simulink model "p1"  (R2014a)
settings: Solver=ode1  SolverMode=SingleTasking  StartTime=0  StopTime=36000  FixedStep=Ts  RelTol=1e-3
PreLoadFcn:
  | InitModel
  | make
InitFcn:
  | InitModel
  | make
values from neighbouring files (symbols this model uses):
  num = num+MTnum(m)    [Build_MtMuMy.m]
  Ts = 0.002    [DSC_Control_Analysis.m]    (also in DSC_Control_Analysis_Exp.m; DSC_Speed_Control_Analysis.m; EC_params_nissan.m; Ext_MPCPara.m = SSD.Ts)
undefined symbols (not defined in the file or in its folder): den, DiscIntNeverNeededParam, gpsins, hal_filter_den, hal_filter_num, Igain_l, Igain_r, Imax_l, Imax_r, Ioff_l, Ioff_r, KB, Kd, KF, Ki, KJ, Kp, param, sglu, wc
libraries: simulink x8, UserBlocks x2, HardwareIO x1, slrtlib x1
(part 2 of 2)

== system p1/Sensor Data and Estimation/Nonlinear Observer/Steering Torque Components/Steering Geometry Calculation ==
  Motor Angles : Inport
  Bus Creator : BusCreator  Inputs=2
  Bus Creator1 : BusCreator  Inputs=2
  Bus Selector1 : BusSelector  OutputSignals=Left,Right
  Left Steer Angle Look-up : Lookup_n-D  NumberOfTableDimensions=1  BreakpointsForDimension1=sglu.fl.sa  Table=sglu.fl.ja  InternalRulePriority=Speed  SaturateOnIntegerOverflow=on  InputSameDT=on
  Left Steer Angle Look-up1 : Lookup_n-D  NumberOfTableDimensions=1  BreakpointsForDimension1=sglu.fl.sa  Table=sglu.fl.mt  InternalRulePriority=Speed  SaturateOnIntegerOverflow=on  InputSameDT=on
  Right Steer Angle Look-up : Lookup_n-D  NumberOfTableDimensions=1  BreakpointsForDimension1=sglu.fr.sa  Table=sglu.fr.ja  InternalRulePriority=Speed  SaturateOnIntegerOverflow=on  InputSameDT=on
  Right Steer Angle Look-up1 : Lookup_n-D  NumberOfTableDimensions=1  BreakpointsForDimension1=sglu.fr.sa  Table=sglu.fr.mt  InternalRulePriority=Speed  SaturateOnIntegerOverflow=on  InputSameDT=on
  Jacking Arm Lengths : Outport
  Mechanical Trails : Outport  Port=2
  wires:
  Motor Angles/1 -> Bus Selector1/1
  Bus Creator/1 -> Jacking Arm Lengths/1
  Left Steer Angle Look-up/1 -> Bus Creator/1  "Left"
  Right Steer Angle Look-up/1 -> Bus Creator/2  "Right"
  Bus Creator1/1 -> Mechanical Trails/1
  Left Steer Angle Look-up1/1 -> Bus Creator1/1  "Left"
  Bus Selector1/1 -> Left Steer Angle Look-up/1, Left Steer Angle Look-up1/1  "<Left>"
  Bus Selector1/2 -> Right Steer Angle Look-up/1, Right Steer Angle Look-up1/1  "<Right>"
  Right Steer Angle Look-up1/1 -> Bus Creator1/2  "Right"

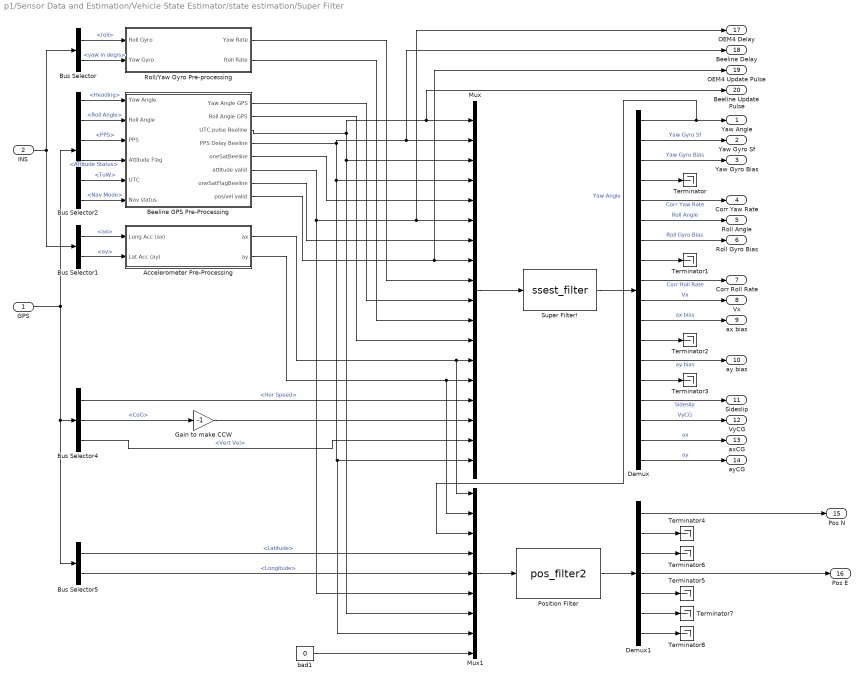
== system p1/Sensor Data and Estimation/Vehicle State Estimator/state estimation/Super Filter ==
  GPS : Inport
  INS : Inport  Port=2
  Accelerometer Pre-Processing : Subsystem
  Beeline GPS Pre-Processing : Subsystem
      mask init:
      | % this code sets the max delay to the value
      | % in ssest_params or to 1000000x that value
      | % if we're in pre-recorded data mode
      | 
      | flag=sum(strcmp(find_system(gcs),[gcs '/Pre-recorded Data']));
      | 
      | if flag==1; % this is pre-recorded mode, set 1000000x larger delay
      |     set_param([gcb '/Delay function'],'Parameters','gpsins.maxbeelinedelayoffline, Ts')
      | else;
      |     set_param([gcb '/Delay function'],'Parameters','gpsins.maxbeelinedelay, Ts')
      | end;
  Bus Selector : BusSelector  OutputSignals=roll,yaw in deg/s
  Bus Selector1 : BusSelector  OutputSignals=ax,ay
  Bus Selector2 : BusSelector  OutputSignals=Heading,Roll Angle,PPS,Attitude Status,ToW,Nav Mode
  Bus Selector4 : BusSelector  OutputSignals=Hor Speed,CoG,Vert Vel
  Bus Selector5 : BusSelector  OutputSignals=Latitude,Longitude
  Demux : Demux  Outputs=[1 1 1 9 1 1 1 4 1 1 1 1 1 16 1 1 1 1]
  Demux1 : Demux  Outputs=[1 1 1 1 1 1 36]
  Gain to make CCW : Gain  Gain=-1
  Mux : Mux  Inputs=18
  Mux1 : Mux  Inputs=9
  Position Filter : S-Function  FunctionName=pos_filter2  Parameters=gpsins.initPosE, gpsins.initPosN  EnableBusSupport=off
  Roll/Yaw Gyro Pre-processing : Subsystem
  Super Filter! : S-Function  FunctionName=ssest_filter  Parameters=gpsins.init_state_hdg, gpsins.init_cov_hdg, gpsins.init_state_roll, gpsins.init_cov_roll, gpsins.init_state_vel, gpsins.init_cov_vel, gpsins.hdgfilter.sens_var, gpsins.hdgfilter.timeconst1, gpsins.hdgfilter.timeconst2, gpsins.hdgfilter.msr_var, gpsins.hdgfilter.init_sf_var, gpsins.diff_yaw, gpsins.rollfilter.sens_var, gpsins.rollfilter.timeconst, gpsins.rollfilter.msr_var, gpsins.diff_roll, gpsins.splitbeelinedelay, gpsins.dist_sensor, gpsins.height_sensor, gpsins.h_gps_ant, gpsins.l_gps_ant, gpsins.velfilter.sens1_var, gpsins.velfilter.sens2_var, gpsins.velfilter.timeconst1, gpsins.velfilter.timeconst2, gpsins.velfilter.msr1_var, gpsins.velfilter.msr2_var, gpsins.diff_vel_x, gpsins.diff_vel_y, gpsins.num_grade_avg, Ts  EnableBusSupport=off
  Terminator{,1..8} (9 alike) : Terminator
  bad1 : Constant  Value=0
  Yaw Angle : Outport
  Yaw Gyro Sf : Outport  Port=2
  Yaw Gyro Bias : Outport  Port=3
  Corr Yaw Rate : Outport  Port=4
  Roll Angle : Outport  Port=5
  Roll Gyro Bias : Outport  Port=6
  Corr Roll Rate : Outport  Port=7
  Vx : Outport  Port=8
  ax bias : Outport  Port=9
  ay bias : Outport  Port=10
  Sideslip : Outport  Port=11
  VyCG : Outport  Port=12
  axCG : Outport  Port=13
  ayCG : Outport  Port=14
  Pos N : Outport  Port=15
  Pos E : Outport  Port=16
  OEM4 Delay : Outport  Port=17
  Beeline Delay : Outport  Port=18
  OEM4 Update Pulse : Outport  Port=19
  Beeline Update Pulse : Outport  Port=20
  wires:
  Beeline GPS Pre-Processing/3(UTC pulse Beeline) -> Mux1/7, Mux/3, Mux/1, Beeline Update Pulse/1
  Beeline GPS Pre-Processing/5(oneSatBeeline) -> Mux/5
  Beeline GPS Pre-Processing/6(attitude valid) -> Mux1/6, OEM4 Delay/1, Mux/6
  Beeline GPS Pre-Processing/7(oneSatFlagBeeline) -> Mux/7
  Roll/Yaw Gyro Pre-processing/1(Yaw Rate) -> Mux/9
  Beeline GPS Pre-Processing/1(Yaw Angle GPS) -> Mux/10
  Roll/Yaw Gyro Pre-processing/2(Roll Rate) -> Mux/11
  Beeline GPS Pre-Processing/2(Roll Angle GPS) -> Mux/12
  Accelerometer Pre-Processing/1(ax) -> Mux/13, Mux1/1
  Accelerometer Pre-Processing/2(ay) -> Mux/14, Mux1/2
  Mux/1 -> Super Filter!/1
  Super Filter!/1 -> Demux/1
  Demux/1 -> Yaw Angle/1, Mux1/3  "Yaw Angle"
  Demux/2 -> Yaw Gyro Sf/1  "Yaw Gyro Sf"
  Demux/3 -> Yaw Gyro Bias/1  "Yaw Gyro Bias"
  Demux/4 -> Terminator/1
  Demux/5 -> Corr Yaw Rate/1  "Corr Yaw Rate"
  Demux/6 -> Roll Angle/1  "Roll Angle"
  Demux/7 -> Roll Gyro Bias/1  "Roll Gyro Bias"
  Demux/8 -> Terminator1/1
  Demux/9 -> Corr Roll Rate/1  "Corr Roll Rate"
  Demux/10 -> Vx/1  "Vx"
  Demux/11 -> ax bias/1  "ax bias"
  Demux/12 -> Terminator2/1
  Demux/13 -> ay bias/1  "ay bias"
  Demux/14 -> Terminator3/1
  Demux/15 -> Sideslip/1  "Sideslip"
  Demux/16 -> VyCG/1  "VyCG"
  Demux/17 -> axCG/1  "ax"
  Demux/18 -> ayCG/1  "ay"
  Mux1/1 -> Position Filter/1
  Position Filter/1 -> Demux1/1
  Demux1/2 -> Terminator4/1
  Demux1/3 -> Terminator6/1
  Demux1/5 -> Terminator5/1
  Demux1/6 -> Terminator7/1
  Demux1/7 -> Terminator8/1
  INS/1 -> Bus Selector/1, Bus Selector1/1
  Bus Selector/1 -> Roll/Yaw Gyro Pre-processing/1(Roll Gyro)  "<roll>"
  Bus Selector/2 -> Roll/Yaw Gyro Pre-processing/2(Yaw Gyro)  "<yaw in deg/s>"
  Bus Selector1/1 -> Accelerometer Pre-Processing/1(Long Acc (ax))  "<ax>"
  Bus Selector1/2 -> Accelerometer Pre-Processing/2(Lat Acc (ay))  "<ay>"
  GPS/1 -> Bus Selector2/1, Bus Selector5/1, Bus Selector4/1
  Bus Selector2/1 -> Beeline GPS Pre-Processing/1(Yaw Angle)  "<Heading>"
  Bus Selector2/2 -> Beeline GPS Pre-Processing/2(Roll Angle)  "<Roll Angle>"
  Bus Selector2/3 -> Beeline GPS Pre-Processing/3("PPS ")  "<PPS>"
  Bus Selector2/4 -> Beeline GPS Pre-Processing/4(Attitude Flag)  "<Attitude Status>"
  Bus Selector2/5 -> Beeline GPS Pre-Processing/5(UTC)  "<ToW>"
  Bus Selector4/1 -> Mux/15  "<Hor Speed>"
  Bus Selector4/2 -> Gain to make CCW/1  "<CoG>"
  Bus Selector4/3 -> Mux/17  "<Vert Vel>"
  Bus Selector5/1 -> Mux1/4  "<Latitude>"
  Bus Selector5/2 -> Mux1/5  "<Longitude>"
  Gain to make CCW/1 -> Mux/16
  Demux1/1 -> Pos N/1
  Demux1/4 -> Pos E/1
  Bus Selector2/6 -> Beeline GPS Pre-Processing/6(Nav status)  "<Nav Mode>"
  Beeline GPS Pre-Processing/8(pos/vel valid) -> OEM4 Update Pulse/1, Mux/8
  Beeline GPS Pre-Processing/4(PPS Delay Beeline) -> Mux1/8, Mux/18, Mux/4, Mux/2, Beeline Delay/1
  bad1/1 -> Mux1/9

== system p1/Sensor Data and Estimation/Vehicle State Estimator/state estimation/Super Filter/Accelerometer Pre-Processing ==
  Long Acc (ax) : Inport
  Lat Acc (ay) : Inport  Port=2
  Memory : Memory
  Sum2 : Sum  Inputs=|++  SaturateOnIntegerOverflow=on  InputSameDT=on  OutDataTypeStr=Inherit: Same as first input
  Sum3 : Sum  Inputs=|++  SaturateOnIntegerOverflow=on  InputSameDT=on  OutDataTypeStr=Inherit: Same as first input
  Sum4 : Sum  Inputs=|+-  SaturateOnIntegerOverflow=on  InputSameDT=on  OutDataTypeStr=Inherit: Same as first input
  Sum5 : Sum  Inputs=|+-  SaturateOnIntegerOverflow=on  InputSameDT=on  OutDataTypeStr=Inherit: Same as first input
  ax Bias : Constant  Value=gpsins.long_acc_bias
  ax sf : Gain  Gain=gpsins.long_acc_sf  SaturateOnIntegerOverflow=on  OutDataTypeStr=Inherit: Same as input  ParamDataTypeStr=Inherit: Same as input
  ay Bias : Constant  Value=gpsins.lat_acc_bias
  ay sf : Gain  Gain=gpsins.lat_acc_sf  SaturateOnIntegerOverflow=on  OutDataTypeStr=Inherit: Same as input  ParamDataTypeStr=Inherit: Same as input
  cross coupling from ax : Gain  Gain=gpsins.long_to_lat  SaturateOnIntegerOverflow=on  OutDataTypeStr=Inherit: Same as input  ParamDataTypeStr=Inherit: Same as input
  cross coupling from ay : Gain  Gain=gpsins.lat_to_long  SaturateOnIntegerOverflow=on  OutDataTypeStr=Inherit: Same as input  ParamDataTypeStr=Inherit: Same as input
  ax : Outport
  ay : Outport  Port=2
  wires:
  Memory/1 -> cross coupling from ax/1
  Sum4/1 -> Memory/1, ax/1
  Sum5/1 -> cross coupling from ay/1, ay/1
  ay sf/1 -> Sum5/1
  cross coupling from ax/1 -> Sum5/2
  ax sf/1 -> Sum4/1
  cross coupling from ay/1 -> Sum4/2
  Long Acc (ax)/1 -> Sum3/1
  Sum3/1 -> ax sf/1
  ax Bias/1 -> Sum3/2
  Sum2/1 -> ay sf/1
  Lat Acc (ay)/1 -> Sum2/1
  ay Bias/1 -> Sum2/2

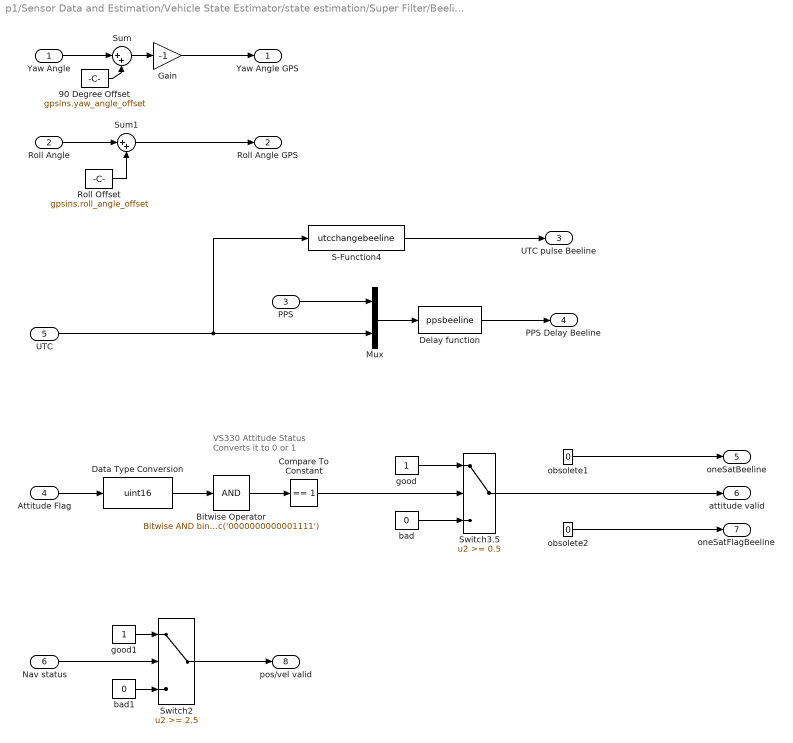
== system p1/Sensor Data and Estimation/Vehicle State Estimator/state estimation/Super Filter/Beeline GPS Pre-Processing ==
  note: VS330 Attitude Status
      | Converts it to 0 or 1
  Yaw Angle : Inport
  Roll Angle : Inport  Port=2
  "PPS " : Inport  Port=3
  Attitude Flag : Inport  Port=4
  UTC : Inport  Port=5
  Nav status : Inport  Port=6
  90 Degree Offset : Constant  Value=gpsins.yaw_angle_offset
  Bitwise Operator : simulink/Logic and Bit Operations/Bitwise Operator  logicop=AND  UseBitMask=on  BitMask=bin2dec('0000000000001111')  BitMaskRealWorld=Stored Integer
  Compare To Constant : simulink/Logic and Bit Operations/Compare To Constant  relop===  const=1  OutDataTypeStr=boolean
  Data Type Conversion : DataTypeConversion  OutDataTypeStr=uint16
  Delay function : S-Function  FunctionName=ppsbeeline  Parameters=gpsins.maxbeelinedelay, Ts  EnableBusSupport=off
  Gain : Gain  Gain=-1  SaturateOnIntegerOverflow=on  OutDataTypeStr=Inherit: Same as input  ParamDataTypeStr=Inherit: Same as input
  Mux : Mux  Inputs=2
  Roll Offset : Constant  Value=gpsins.roll_angle_offset
  S-Function4 : S-Function  FunctionName=utcchangebeeline  Parameters=Ts  EnableBusSupport=off
  Sum : Sum  Inputs=|++  SaturateOnIntegerOverflow=on  InputSameDT=on  OutDataTypeStr=Inherit: Same as first input
  Sum1 : Sum  Inputs=|++  SaturateOnIntegerOverflow=on  InputSameDT=on  OutDataTypeStr=Inherit: Same as first input
  Switch2 : Switch  Threshold=2.5  SaturateOnIntegerOverflow=on  InputSameDT=on
  Switch3.5 : Switch  Threshold=0.5  SaturateOnIntegerOverflow=on  InputSameDT=on
  bad : Constant  Value=0
  bad1 : Constant  Value=0
  good : Constant
  good1 : Constant
  obsolete1 : Constant  Value=0
  obsolete2 : Constant  Value=0
  Yaw Angle GPS : Outport
  Roll Angle GPS : Outport  Port=2
  UTC pulse Beeline : Outport  Port=3
  PPS Delay Beeline : Outport  Port=4
  oneSatBeeline : Outport  Port=5
  attitude valid : Outport  Port=6
  oneSatFlagBeeline : Outport  Port=7
  pos/vel valid : Outport  Port=8
  wires:
  Roll Offset/1 -> Sum1/2
  Sum1/1 -> Roll Angle GPS/1
  Roll Angle/1 -> Sum1/1
  Yaw Angle/1 -> Sum/1
  Sum/1 -> Gain/1
  90 Degree Offset/1 -> Sum/2
  bad/1 -> Switch3.5/3
  good/1 -> Switch3.5/1
  S-Function4/1 -> UTC pulse Beeline/1
  Delay function/1 -> PPS Delay Beeline/1
  "PPS "/1 -> Mux/1
  UTC/1 -> S-Function4/1, Mux/2
  Mux/1 -> Delay function/1
  obsolete2/1 -> oneSatFlagBeeline/1
  obsolete1/1 -> oneSatBeeline/1
  Gain/1 -> Yaw Angle GPS/1
  Attitude Flag/1 -> Data Type Conversion/1
  Data Type Conversion/1 -> Bitwise Operator/1
  Bitwise Operator/1 -> Compare To Constant/1
  Compare To Constant/1 -> Switch3.5/2
  bad1/1 -> Switch2/3
  good1/1 -> Switch2/1
  Nav status/1 -> Switch2/2
  Switch2/1 -> pos/vel valid/1
  Switch3.5/1 -> attitude valid/1

== system p1/Sensor Data and Estimation/Vehicle State Estimator/state estimation/Super Filter/Roll//Yaw Gyro Pre-processing ==
  Roll Gyro : Inport
  Yaw Gyro : Inport  Port=2
  Memory : Memory
  Roll Gyro Bias : Constant  Value=gpsins.roll_rate_bias
  Sum2 : Sum  Inputs=|++  SaturateOnIntegerOverflow=on  InputSameDT=on  OutDataTypeStr=Inherit: Same as first input
  Sum3 : Sum  Inputs=|+-  SaturateOnIntegerOverflow=on  InputSameDT=on  OutDataTypeStr=Inherit: Same as first input
  Sum4 : Sum  Inputs=|++  SaturateOnIntegerOverflow=on  InputSameDT=on  OutDataTypeStr=Inherit: Same as first input
  Sum5 : Sum  Inputs=|+-  SaturateOnIntegerOverflow=on  InputSameDT=on  OutDataTypeStr=Inherit: Same as first input
  Yaw Gyro Bias : Constant  Value=gpsins.yaw_rate_bias
  cross coupling from roll : Gain  Gain=gpsins.roll_to_yaw  SaturateOnIntegerOverflow=on  OutDataTypeStr=Inherit: Same as input  ParamDataTypeStr=Inherit: Same as input
  cross coupling from yaw : Gain  Gain=gpsins.yaw_to_roll  SaturateOnIntegerOverflow=on  OutDataTypeStr=Inherit: Same as input  ParamDataTypeStr=Inherit: Same as input
  roll rate sf : Gain  Gain=gpsins.roll_rate_sf  SaturateOnIntegerOverflow=on  OutDataTypeStr=Inherit: Same as input  ParamDataTypeStr=Inherit: Same as input
  yaw rate sf : Gain  SaturateOnIntegerOverflow=on  OutDataTypeStr=Inherit: Same as input  ParamDataTypeStr=Inherit: Same as input
  Yaw Rate : Outport
  Roll Rate : Outport  Port=2
  wires:
  Memory/1 -> cross coupling from roll/1
  Sum3/1 -> Memory/1, Roll Rate/1
  Sum5/1 -> cross coupling from yaw/1, Yaw Rate/1
  roll rate sf/1 -> Sum3/1
  yaw rate sf/1 -> Sum5/1
  cross coupling from roll/1 -> Sum5/2
  cross coupling from yaw/1 -> Sum3/2
  Sum4/1 -> roll rate sf/1
  Roll Gyro/1 -> Sum4/2
  Roll Gyro Bias/1 -> Sum4/1
  Yaw Gyro Bias/1 -> Sum2/2
  Sum2/1 -> yaw rate sf/1
  Yaw Gyro/1 -> Sum2/1
